simulink model "equlibrium"  (Simulink 7.4)
settings: Solver=ode3  StartTime=0.0  StopTime=5  FixedStep=0.01  RelTol=1e-3
values from neighbouring files (symbols this model uses):
  A = [0,1; g/l,0]    [in.m]
  b = [0;-1/m/l/l]    [in.m]
  c = [1,0;0,1]    [in.m]
  cn = [1,0;0,0]    [in.m]
  k = (place(A,b,p))    [in.m]
  l = (place(A',cn',p))'    [in.m]
  th0 = 5    [in.m]
  v0 = 3    [in.m]
settings Model: Creator=Admin  LastModifiedBy=my comp

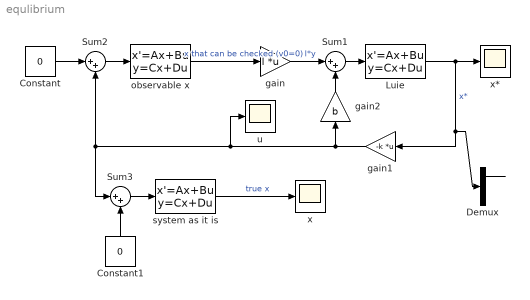
== system equlibrium ==
  Constant : Constant  Value=0  OutDataType=fixdt(1, 16)  OutScaling=2^0
  Constant1 : Constant  Value=0  OutDataType=fixdt(1, 16)  OutScaling=2^0
  Demux : Demux  Outputs=2
  Luie : StateSpace  A=A-l*c  B=eye(2)  C=eye(2)  D=zeros(2)  X0=[th0 0]
  Sum1 : Sum  Inputs=|++  OutDataType=fixdt(1, 16)  OutScaling=2^0
  Sum2 : Sum  Inputs=|++  OutDataType=fixdt(1, 16)  OutScaling=2^0
  Sum3 : Sum  Inputs=|++  OutDataType=fixdt(1, 16)  OutScaling=2^0
  gain : Gain  Gain=l  Multiplication=Matrix(K*u) (u vector)  ParameterDataType=fixdt(1, 16)  ParameterScaling=2^0  OutDataType=fixdt(1, 16)  OutScaling=2^0
  gain1 : Gain  Gain=-k  Multiplication=Matrix(K*u) (u vector)  ParameterDataType=fixdt(1, 16)  ParameterScaling=2^0  OutDataType=fixdt(1, 16)  OutScaling=2^0
  gain2 : Gain  Gain=b  ParameterDataType=fixdt(1, 16)  ParameterScaling=2^0  OutDataType=fixdt(1, 16)  OutScaling=2^0
  observable x : StateSpace  A=A  B=b  C=cn  D=[0;0]  X0=[th0 v0]
  system as it is : StateSpace  A=A  B=b  C=[1,0;0,1]  D=[0;0]  X0=[th0 v0]
  u : Scope
      settings: TimeRange=5  YMin=-7e+027  YMax=0
  x : Scope
      settings: TimeRange=5  YMin=-0.6000000000000001  YMax=0.3999999999999999
  x* : Scope
      settings: TimeRange=5  YMin=-0.6000000000000001  YMax=0.3999999999999999  SaveName=ScopeData3
  wires:
  system as it is/1 -> x/1  "true x"
  Luie/1 -> x*/1, gain1/1, Demux/1  "x*"
  Sum1/1 -> Luie/1
  observable x/1 -> gain/1  "x that can be checked (v0=0)"
  gain/1 -> Sum1/1  "l*y"
  Sum2/1 -> observable x/1
  Sum3/1 -> system as it is/1
  gain1/1 -> gain2/1, u/1, Sum2/2, Sum3/1
  gain2/1 -> Sum1/2
  Constant/1 -> Sum2/1
  Constant1/1 -> Sum3/2
  Demux/1 -> ?
